simulink model "Off-grid PV design simulink"  (R2023b)
settings: Solver=ode23t  StartTime=0.0  StopTime=0.5  RelTol=1e-3
undefined symbols (not defined in the file): Acid, Lead
libraries: spsSeriesRLCBranchLib x5, spsIGBTDiodeLib x4, spsVoltageMeasurementLib x3, simulink x2, spsBatteryLib x1, spsDiodeLib x1, spsMeanLib x1, spsPWMGeneratorDCDCLib x1, spsMosfetLib x1, spsPVArrayLib x1, spsSeriesRLCLoadLib x1, spsVariableRatioTransformerLib x1
settings Model: Creator=Anl  LastModifiedBy=uthay
settings SolverCC: AlgebraicLoopSolver=TrustRegion
settings DebuggingCC: UnconnectedInputMsg=warning  UnconnectedOutputMsg=warning  UnconnectedLineMsg=warning
settings ModelReferenceCC: EnableRefExpFcnMdlSchedulingChecks=on
settings RTWCC: DLArmComputeVersion=19.05

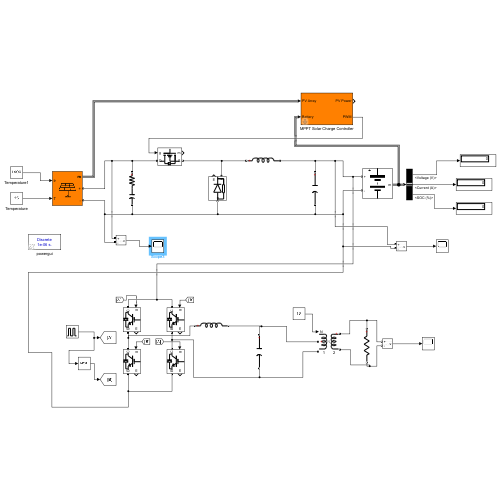
[thumbnail: Simulink's stored preview of the top-level diagram]
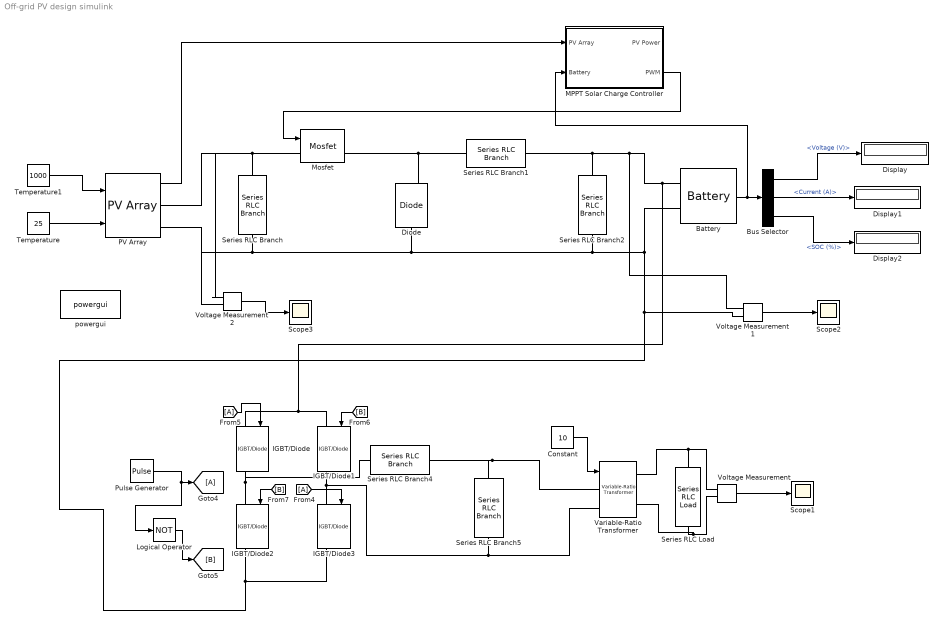
== system Off-grid PV design simulink ==
  Battery : spsBatteryLib/Battery  BatType=Lead-Acid  ShowTempParam=off  ThermalPreset=no  ShowAgeParam=off  NomV=24  NomQ=4096  SOC=20  Batt_Tr=1  PresetModel=on  MaxQ=4266.6667  MinV=18  FullV=26.1316  Dis_rate=819.2  R=5.8594e-05  Normal_OP=1270.8978  expZone="[24.4342      13.6533]"  current=[6.5 13 32.5]  Units=Time  Tci=20  NomT=20  T2=-30  MaxQ2=4.8  FullV2=7.1  Normal_OP2=5.655  expZone2="[6.58           1]"  Rca=0.6  ti=2000  Dp=0  Neq0=0  Tsim=1e6  Ta1=25  Qeol=5.4*0.9  Reol=0.013333*1.2  Char_age=[2.3478, 3]  Dis_age=[2.3478, 10]  N1=1500  N2=10500  N3=1000  N4=1400  Ta2=45  N5=950
      settings: LibrarySourceBlock=electricdrivelib/Extra Sources/Battery
  Bus Selector : BusSelector  OutputSignals=Voltage (V),Current (A),SOC (%)
  Constant : Constant  Value=10
  Diode : spsDiodeLib/Diode  Ron=0.001  Lon=0  Vf=0.8  IC=0  UseSnubber=0  Rs=500  Cs=250e-9  Measurements=on
  Display : Display
  Display1 : Display
  Display2 : Display
  From4 : From
  From5 : From
  Goto4 : Goto
  IGBT/Diode{,1..3} (4 alike) : spsIGBTDiodeLib/IGBT//Diode  Ron=1e-3  Rs=1e5  Cs=inf  Measurements=on
  Logical Operator : Logic  Operator=NOT  AllPortsSameDT=off  OutDataTypeStr=boolean
  MPPT Solar Charge Controller : Subsystem  mask(MPPT Solar Charge Controller Block){dD=125e-6, BattCV=24, Fsw=10000}
      mask prompts: dD "MPPT Duty Cycle (delta) Step Size"; BattCV "Battery Charging Constant Voltage (V)"; Fsw "PWM Switching frequency (Hz):"
      mask help:
      | MPPT Solar Charge Controller Block
      | Developed by Rodney Tan (PhD)
      | Version 1.00 Oct 2019
      |
      | This block perform solar photovoltaic Maximum Power Point Tracking based on Perturbation & Observation algorithm and charge lead acid battery using three stage charging algorithm.
      mask Help:
      | <b><u>Block Setting</u></b>
      | 
      | <b>MPPT Duty Cycle Step Size</b>
      | Specify the MPPT duty cycle (delta) step size. Default value is 1e-5.
      | 
      | <b>Battery Charging Constant Voltage (V)</b>
      | Specify the battery charging constant voltage for absorption stage.
      | 
      | <b>PWM Switching Frequency (Hz)</b>
      | Specify the PWM switching frequency in Hz.
      mask TypeOptions Fsw:
      | PWM Generator
      | (DC-DC)/Fsw
  Mosfet : spsMosfetLib/Mosfet  Ron=0.1  Lon=0  Rd=0.01  Vfd=0  IC=0  Rs=1e5  Cs=inf  Measurements=on
  PV Array : spsPVArrayLib/PV Array  Npar=3  Nser=1  PlotType=array @ 25 deg.C & specified irradiances  S_vec="[ 1000  500  100 ]"  Temp_C_vec="[ 45 25  ]"  ModuleName=User-defined  PlotWhenSelected=off  Pm=335.58  Ncell=72  Voc=41.5  Isc=10.36  Vm=34  Im=9.87  beta_Voc_pc=-0.28  alpha_Isc_pc=0.048  beta_Voc=-0.1162  alpha_Isc=0.0049728  IL=10.5776  I0=1.5092e-11  nI=0.82328  Rsh=154.3518  Rs=0.28403  RobustModel=off  RobustCellTemperature=313.3991  BAL=on  Tc=1e-6  Tfilter=5e-5
  Pulse Generator : DiscretePulseGenerator  PulseType=Time based  Period=0.02  PulseWidth=50
  Scope1 : Scope
  Scope2 : Scope
  Scope3 : Scope
  Series RLC Branch : spsSeriesRLCBranchLib/Series RLC Branch  LConnTagsString=__new0  RConnTagsString=__new0  BranchType=RC  Resistance=0.0001  Inductance=1e-3  SetiL0=off  InitialCurrent=0  Capacitance=1000e-6  Setx0=off  InitialVoltage=0  Measurements=None
  Series RLC Branch1 : spsSeriesRLCBranchLib/Series RLC Branch  LConnTagsString=__new0  RConnTagsString=__new0  BranchType=L  Resistance=1  Inductance=3.3e-3  SetiL0=off  InitialCurrent=0  Capacitance=1e-6  Setx0=off  InitialVoltage=0  Measurements=None
  Series RLC Branch2 : spsSeriesRLCBranchLib/Series RLC Branch  LConnTagsString=__new0  RConnTagsString=__new0  BranchType=C  Resistance=364  Inductance=0.783e-3  SetiL0=off  InitialCurrent=0  Capacitance=0.26e-6  Setx0=off  InitialVoltage=0  Measurements=None
  Series RLC Branch4 : spsSeriesRLCBranchLib/Series RLC Branch  LConnTagsString=__new0  RConnTagsString=__new0  BranchType=L  Resistance=1  Inductance=0.002  SetiL0=off  InitialCurrent=0  Capacitance=0.006  Setx0=off  InitialVoltage=0  Measurements=None
  Series RLC Branch5 : spsSeriesRLCBranchLib/Series RLC Branch  LConnTagsString=__new0  RConnTagsString=__new0  BranchType=C  Resistance=1  Inductance=1e-3  SetiL0=off  InitialCurrent=0  Capacitance=0.0065  Setx0=off  InitialVoltage=0  Measurements=None
  Series RLC Load : spsSeriesRLCLoadLib/Series RLC Load  LConnTagsString=a  RConnTagsString=__new0  NominalVoltage=230  NominalFrequency=50  ActivePower=1000  InductivePower=0  CapacitivePower=0  Setx0=off  InitialVoltage=0  SetiL0=off  InitialCurrent=0  Measurements=None  LoadType=constant Z
  Temperature : Constant  Value=25
  Temperature1 : Constant  Value=1000
  Variable-Ratio Transformer : spsVariableRatioTransformerLib/Variable-Ratio Transformer
  Voltage Measurement : spsVoltageMeasurementLib/Voltage Measurement  PhasorSimulation=off  OutputType=Complex  PSBequivalent=0
  Voltage Measurement1 : spsVoltageMeasurementLib/Voltage Measurement  PhasorSimulation=off  OutputType=Complex  PSBequivalent=0
  Voltage Measurement2 : spsVoltageMeasurementLib/Voltage Measurement  PhasorSimulation=off  OutputType=Complex  PSBequivalent=0
  powergui : sps_lib/powergui  Priority=1  SimulationMode=Discrete  SampleTime=1e-6  frequency=60  Iterations=50  frequencyindice=0  Pbase=100e6  ErrMax=1e-4  UnitsV=kV  UnitsW=MW  buscounter=0  FunctionMessages=off  echomessages=off  EnableUseOfTLC=off  CurrentSourceSwitches=off  DisableSnubberDevices=off  DisableRonSwitches=off  DisableVfSwitches=off  DisplayEquations=off  AutomaticDiscreteSolvers=off  SolverType=Tustin/Backward Euler (TBE)  Interpol=off  ExternalGateDelay=off  methode=off  Ts=100  x0status=blocks  SPID=on  SwTol=0  HookPort=off  NonlinearTolerance=1e-4  nMaxIteration=100  ContinueOnMaxIteration=off  RestoreLinks=warning  ResistiveCurrentMeasurement=off  Frange=[0:2:500]  Ylog=off  Xlog=on  ShowGrid=off  save=off  variable=ZData  structure=0  ZoomFFT=off  StartTime=0.0  cycles=1  DisplayStyle=1  fundamental=60  FreqAxis=off  MaxFrequency=1000  frequencyindicesteady=1  RmsSteady=1  display=off
  wires:
  Battery/1 -> MPPT Solar Charge Controller/2(Battery), Bus Selector/1
  PV Array/1 -> MPPT Solar Charge Controller/1(PV Array)
  Temperature/1 -> PV Array/2
  Voltage Measurement/1 -> Scope1/1
  Voltage Measurement1/1 -> Scope2/1
  Voltage Measurement2/1 -> Scope3/1
  Constant/1 -> Variable-Ratio Transformer/1
  [B] -> IGBT/Diode2/1
  Logical Operator/1 -> [B]
  From5/1 -> IGBT/Diode/1
  From4/1 -> IGBT/Diode3/1
  Pulse Generator/1 -> Logical Operator/1, Goto4/1
  [B] -> IGBT/Diode1/1
  Temperature1/1 -> PV Array/1
  Bus Selector/1 -> Display/1  "<Voltage (V)>"
  Bus Selector/2 -> Display1/1  "<Current (A)>"
  MPPT Solar Charge Controller/2(PWM) -> Mosfet/1
  Bus Selector/3 -> Display2/1  "<SOC (%)>"
  connections:
  IGBT/Diode3/RConn1 -- IGBT/Diode2/RConn1 -- Battery/LConn2 -- Series RLC Branch2/RConn1 -- Voltage Measurement2/LConn2 -- PV Array/RConn2 -- Series RLC Branch/RConn1 -- Diode/LConn1 -- Voltage Measurement1/LConn2
  Diode/RConn1 -- Series RLC Branch1/LConn1 -- Mosfet/RConn1
  IGBT/Diode/LConn1 -- IGBT/Diode1/LConn1 -- Voltage Measurement1/LConn1 -- Series RLC Branch2/LConn1 -- Series RLC Branch1/RConn1 -- Battery/LConn1
  Series RLC Branch/LConn1 -- PV Array/RConn1 -- Voltage Measurement2/LConn1 -- Mosfet/LConn1
  Voltage Measurement/LConn2 -- Variable-Ratio Transformer/RConn2 -- Series RLC Load/RConn1
  Voltage Measurement/LConn1 -- Variable-Ratio Transformer/RConn1 -- Series RLC Load/LConn1
  Series RLC Branch5/LConn1 -- Series RLC Branch4/RConn1 -- Variable-Ratio Transformer/LConn1
  IGBT/Diode2/LConn1 -- Series RLC Branch4/LConn1 -- IGBT/Diode/RConn1
  IGBT/Diode3/LConn1 -- Variable-Ratio Transformer/LConn2 -- Series RLC Branch5/RConn1 -- IGBT/Diode1/RConn1

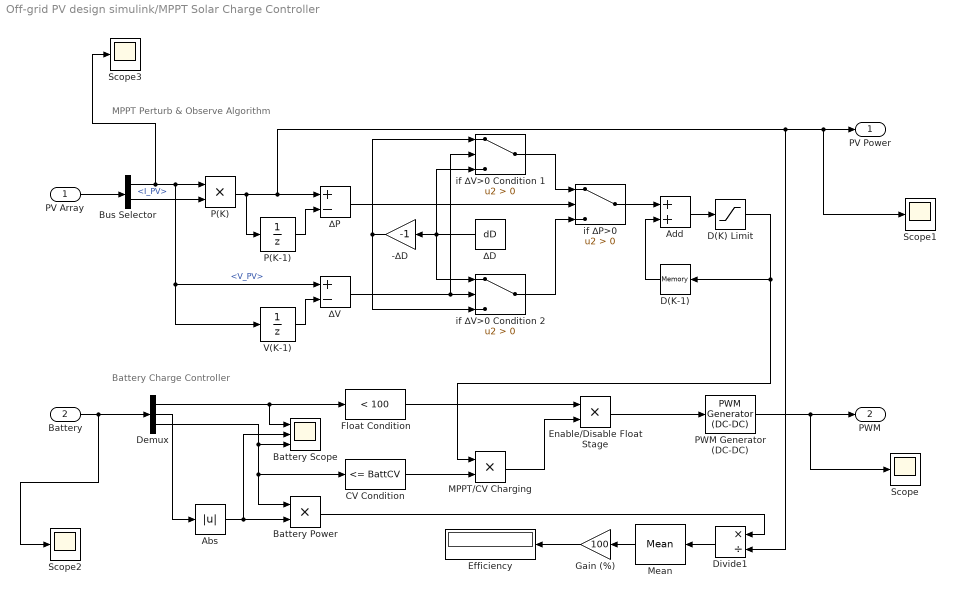
== system Off-grid PV design simulink/MPPT Solar Charge Controller ==
  note: Battery Charge Controller
  note: MPPT Perturb & Observe Algorithm
  PV Array : Inport
  Battery : Inport  Port=2
  -∆D : Gain  Gain=-1
  Abs : Abs  SaturateOnIntegerOverflow=off
  Add : Sum
  Battery Power : Product
  Battery Scope : Scope  NumInputPorts=3
  Bus Selector : BusSelector  OutputSignals=V_PV,I_PV
  CV Condition : simulink/Logic and Bit Operations/Compare To Constant  relop=<=  const=BattCV  OutDataTypeStr=boolean
  D(K) Limit : Saturate  UpperLimit=0.6  LowerLimit=0.4
  D(K-1) : Memory  InitialCondition=0.5  InheritSampleTime=on  LinearizeMemory=on  LinearizeAsDelay=on
  Demux : Demux  Outputs=3
  Divide1 : Product  Inputs=*/
  Efficiency : Display
  Enable/Disable Float Stage : Product
  Float Condition : simulink/Logic and Bit Operations/Compare To Constant  relop=<  const=100  OutDataTypeStr=boolean
  Gain (%) : Gain  Gain=100
  MPPT/CV Charging : Product
  Mean : spsMeanLib/Mean  Freq=1  Vinit=0  Ts=0
  P(K) : Product
  P(K-1) : UnitDelay  SampleTime=-1  HasFrameUpgradeWarning=on
  PWM Generator (DC-DC) : spsPWMGeneratorDCDCLib/PWM Generator (DC-DC)  Fsw=Fsw  Ts=0
  Scope{,1..3} (4 alike) : Scope
  V(K-1) : UnitDelay  SampleTime=-1  HasFrameUpgradeWarning=on
  if ∆P>0 : Switch  Criteria=u2 > Threshold  SaturateOnIntegerOverflow=off  InputSameDT=off
  if ∆V>0 Condition 1 : Switch  Criteria=u2 > Threshold  SaturateOnIntegerOverflow=off  InputSameDT=off
  if ∆V>0 Condition 2 : Switch  Criteria=u2 > Threshold  SaturateOnIntegerOverflow=off  InputSameDT=off
  ∆D : Constant  Value=dD
  ∆P : Sum  Inputs=+-
  ∆V : Sum  Inputs=+-
  PV Power : Outport  VectorParamsAs1DForOutWhenUnconnected=off
  PWM : Outport  Port=2  VectorParamsAs1DForOutWhenUnconnected=off
  wires:
  if ∆V>0 Condition 1/1 -> if ∆P>0/1
  ∆P/1 -> if ∆P>0/2
  P(K-1)/1 -> ∆P/2
  V(K-1)/1 -> ∆V/2
  ∆V/1 -> if ∆V>0 Condition 2/2, if ∆V>0 Condition 1/2
  Add/1 -> D(K) Limit/1
  if ∆V>0 Condition 2/1 -> if ∆P>0/3
  D(K-1)/1 -> Add/2
  ∆D/1 -> if ∆V>0 Condition 2/1, -∆D/1, if ∆V>0 Condition 1/3
  -∆D/1 -> if ∆V>0 Condition 2/3, if ∆V>0 Condition 1/1
  PWM Generator (DC-DC)/1 -> Scope/1, PWM/1
  Enable/Disable Float Stage/1 -> PWM Generator (DC-DC)/1
  Float Condition/1 -> Enable/Disable Float Stage/1
  CV Condition/1 -> MPPT/CV Charging/2
  Battery/1 -> Scope2/1, Demux/1
  Demux/3 -> Battery Scope/3, CV Condition/1, Battery Power/1
  Demux/1 -> Float Condition/1, Battery Scope/1
  MPPT/CV Charging/1 -> Enable/Disable Float Stage/2
  Demux/2 -> Abs/1
  Divide1/1 -> Mean/1
  Mean/1 -> Gain (%)/1
  Abs/1 -> Battery Scope/2, Battery Power/2
  Bus Selector/2 -> P(K)/2  "<I_PV>"
  Battery Power/1 -> Divide1/1
  Bus Selector/1 -> Scope3/1, ∆V/1, V(K-1)/1, P(K)/1  "<V_PV>"
  PV Array/1 -> Bus Selector/1
  if ∆P>0/1 -> Add/1
  D(K) Limit/1 -> D(K-1)/1, MPPT/CV Charging/1
  Gain (%)/1 -> Efficiency/1
  P(K)/1 -> ∆P/1, Divide1/2, Scope1/1, PV Power/1, P(K-1)/1
